simulink model "Pacemaker_Assignment2_group33"  (R2020a)
settings: Solver=FixedStepAuto  StartTime=0.0  StopTime=10.0  FixedStep=1e-3  RelTol=1e-3  EnableMultiTasking=on
undefined symbols (not defined in the file): D0, D1, D10, D11, D12, D13, D2, D3, D4, D5, D6, D7, D8, D9, magnitude, PTA0, PTA1, PTA2, PTB23, PTB9, PTC16, PTC17, PTC2, PTC3, PTC4, PTD0, PTD1, PTD2, PTD3
libraries: frdmk64flib x17, dspstat3 x1
settings Model: ExtModeTrigDuration=5  Creator=sxj  LastModifiedBy=sxj
settings OptimizationCC: EnhancedBackFolding=on  PassReuseOutputArgsAs=Individual arguments  ZeroExternalMemoryAtStartup=off  ZeroInternalMemoryAtStartup=off  MaxStackSize=64  OptimizeBlockOrder=speed  DifferentSizesBufferReuse=on  OptimizationCustomize=off  EfficientTunableParamExpr=on
settings DebuggingCC: ParameterTunabilityLossMsg=error
settings HardwareCC: ProdBitPerPointer=32  ProdBitPerSizeT=32  ProdBitPerPtrDiffT=32  ProdLargestAtomicInteger=Long  ProdLargestAtomicFloat=Double  ProdWordSize=32  ProdHWDeviceType=ARM Compatible->ARM Cortex
settings SFSimCC: MATLABDynamicMemAlloc=off
settings RTWCC: SystemTargetFile=ert.tlc  HardwareBoard=NXP FRDM-K64F  TemplateMakefile=ert_default_tmf  Toolchain=GNU Tools for ARM Embedded Processors
settings CodeAppCC: ForceParamTrailComments=on  IgnoreCustomStorageClasses=off  OperatorAnnotations=on  SimulinkDataObjDesc=on  SFDataObjDesc=on  InsertBlockDesc=on

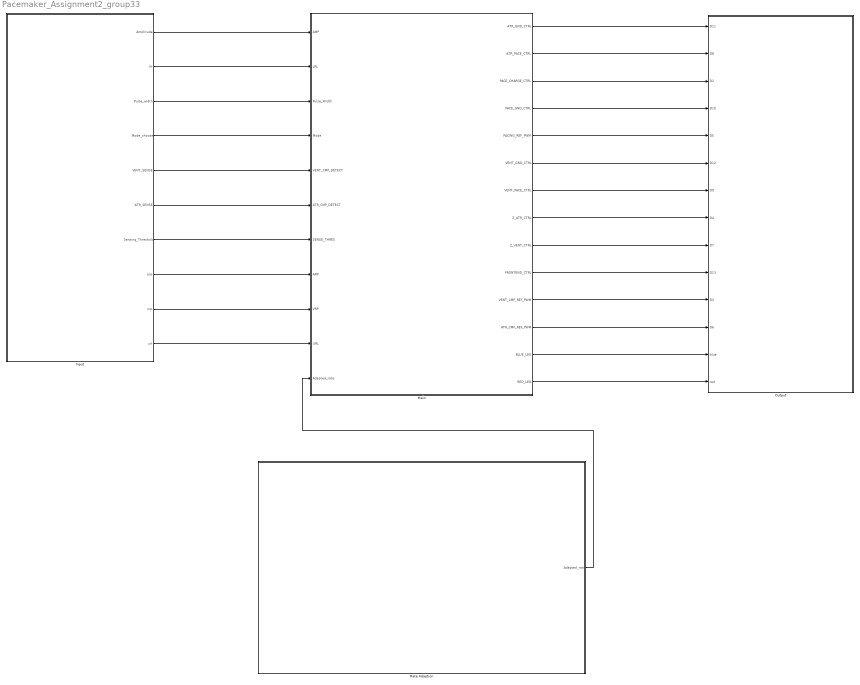
== system Pacemaker_Assignment2_group33 ==
  Input : Subsystem
  Main : Stateflow chart  TreatAsAtomicUnit=on
  Output : Subsystem
  Rate Adaption : Subsystem
  wires:
  Input/1(Amplitude) -> Main/1(AMP)
  Input/2(lrl) -> Main/2(LRL)
  Input/3(Pulse_width) -> Main/3(Pulse_Width)
  Input/4(Mode_choose) -> Main/4(Mode)
  Input/5(VENT_SENSE) -> Main/5(VENT_CMP_DETECT)
  Input/6(ATR_SENSE) -> Main/6(ATR_CMP_DETECT)
  Input/7(Sensing_Threshold) -> Main/7(SENSE_THRES)
  Main/1(ATR_GND_CTRL) -> Output/1(D11)
  Main/2(ATR_PACE_CTRL) -> Output/2(D8)
  Main/3(PACE_CHARGE_CTRL) -> Output/3(D2)
  Main/4(PACE_GND_CTRL) -> Output/4(D10)
  Main/5(PACING_REF_PWM) -> Output/5(D5)
  Main/6(VENT_GND_CTRL) -> Output/6(D12)
  Main/7(VENT_PACE_CTRL) -> Output/7(D9)
  Main/8(Z_ATR_CTRL) -> Output/8(D4)
  Main/9(Z_VENT_CTRL) -> Output/9(D7)
  Main/10(FRONTEND_CTRL) -> Output/10(D13)
  Main/11(VENT_CMP_REF_PWM) -> Output/11(D3)
  Main/12(ATR_CMP_REF_PWM) -> Output/12(D6)
  Main/13(BLUE_LED) -> Output/13(blue)
  Main/14(RED_LED) -> Output/14(red)
  Input/8(arp) -> Main/8(ARP)
  Input/9(vrp) -> Main/9(VRP)
  Input/10(url) -> Main/10(URL)
  Rate Adaption/1(Adapted_rate) -> Main/11(Adapted_rate)

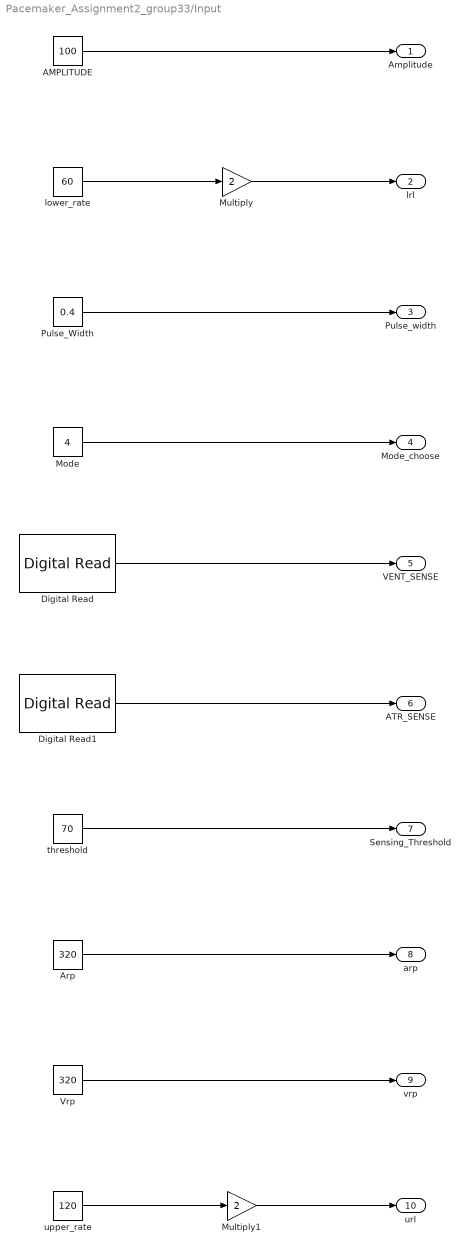
== system Pacemaker_Assignment2_group33/Input ==
  AMPLITUDE : Constant  Value=100
  Arp : Constant  Value=320
  Digital Read : frdmk64flib/Digital Read  Whichpin=PTC17 (D1)  SampleTime=-1
  Digital Read1 : frdmk64flib/Digital Read  Whichpin=PTC16 (D0)  SampleTime=-1
  Mode : Constant  Value=4
  Multiply : Gain  Gain=2
  Multiply1 : Gain  Gain=2
  Pulse_Width : Constant  Value=0.4
  Vrp : Constant  Value=320
  lower_rate : Constant  Value=60
  threshold : Constant  Value=70
  upper_rate : Constant  Value=120
  Amplitude : Outport
  lrl : Outport  Port=2
  Pulse_width : Outport  Port=3
  Mode_choose : Outport  Port=4
  VENT_SENSE : Outport  Port=5
  ATR_SENSE : Outport  Port=6
  Sensing_Threshold : Outport  Port=7
  arp : Outport  Port=8
  vrp : Outport  Port=9
  url : Outport  Port=10
  wires:
  AMPLITUDE/1 -> Amplitude/1
  Pulse_Width/1 -> Pulse_width/1
  Mode/1 -> Mode_choose/1
  Digital Read/1 -> VENT_SENSE/1
  Digital Read1/1 -> ATR_SENSE/1
  threshold/1 -> Sensing_Threshold/1
  Arp/1 -> arp/1
  Vrp/1 -> vrp/1
  lower_rate/1 -> Multiply/1
  Multiply/1 -> lrl/1
  upper_rate/1 -> Multiply1/1
  Multiply1/1 -> url/1

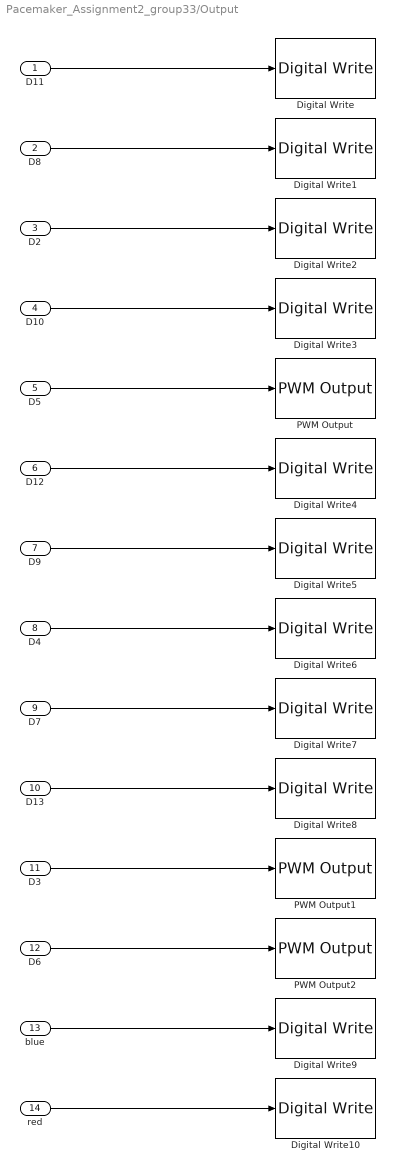
== system Pacemaker_Assignment2_group33/Output ==
  D11 : Inport
  D8 : Inport  Port=2
  D2 : Inport  Port=3
  D10 : Inport  Port=4
  D5 : Inport  Port=5
  D12 : Inport  Port=6
  D9 : Inport  Port=7
  D4 : Inport  Port=8
  D7 : Inport  Port=9
  D13 : Inport  Port=10
  D3 : Inport  Port=11
  D6 : Inport  Port=12
  blue : Inport  Port=13
  red : Inport  Port=14
  Digital Write : frdmk64flib/Digital Write  Whichpin=PTD2 (D11)
  Digital Write1 : frdmk64flib/Digital Write  Whichpin=PTA0 (D8)
  Digital Write10 : frdmk64flib/Digital Write  Whichpin=RED_LED
  Digital Write2 : frdmk64flib/Digital Write  Whichpin=PTB9 (D2)
  Digital Write3 : frdmk64flib/Digital Write  Whichpin=PTD0 (D10)
  Digital Write4 : frdmk64flib/Digital Write  Whichpin=PTD3 (D12)
  Digital Write5 : frdmk64flib/Digital Write  Whichpin=PTC4 (D9)
  Digital Write6 : frdmk64flib/Digital Write  Whichpin=PTB23 (D4)
  Digital Write7 : frdmk64flib/Digital Write  Whichpin=PTC3 (D7)
  Digital Write8 : frdmk64flib/Digital Write  Whichpin=PTD1 (D13)
  Digital Write9 : frdmk64flib/Digital Write  Whichpin=BLUE_LED
  PWM Output : frdmk64flib/PWM Output  Whichpin=PTA2 (D5)  InitialFrequency=2000  InitialDutyCycle=0
  PWM Output1 : frdmk64flib/PWM Output  Whichpin=PTA1 (D3)  InitialFrequency=2000  InitialDutyCycle=0
  PWM Output2 : frdmk64flib/PWM Output  Whichpin=PTC2 (D6)  InitialFrequency=2000  InitialDutyCycle=0
  wires:
  D11/1 -> Digital Write/1
  D8/1 -> Digital Write1/1
  D2/1 -> Digital Write2/1
  D10/1 -> Digital Write3/1
  D5/1 -> PWM Output/1
  D12/1 -> Digital Write4/1
  D9/1 -> Digital Write5/1
  D4/1 -> Digital Write6/1
  D7/1 -> Digital Write7/1
  D13/1 -> Digital Write8/1
  D3/1 -> PWM Output1/1
  D6/1 -> PWM Output2/1
  blue/1 -> Digital Write9/1
  red/1 -> Digital Write10/1

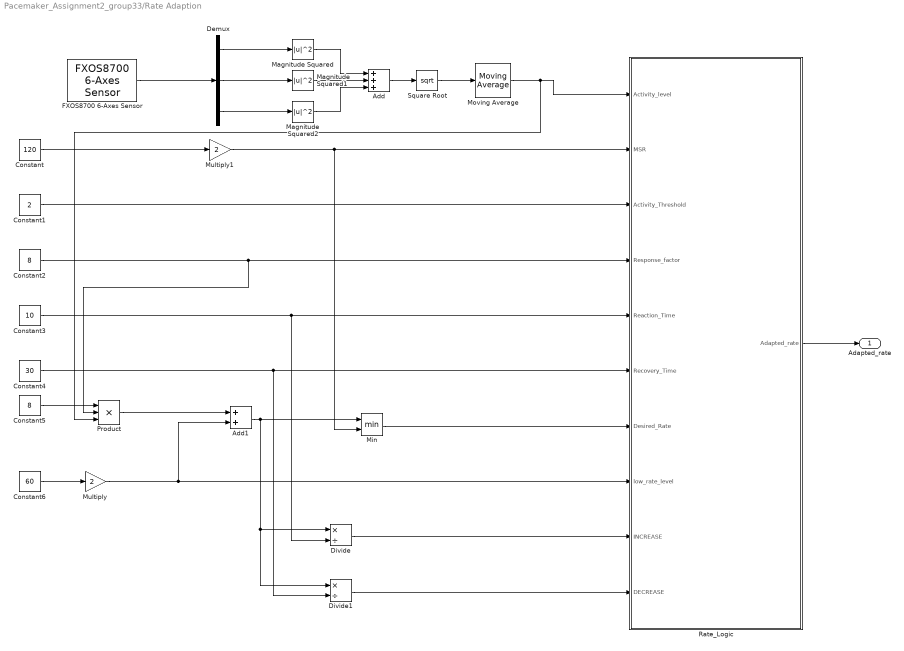
== system Pacemaker_Assignment2_group33/Rate Adaption ==
  Add : Sum  Inputs=+++
  Add1 : Sum
  Constant : Constant  Value=120
  Constant1 : Constant  Value=2
  Constant2 : Constant  Value=8
  Constant3 : Constant  Value=10
  Constant4 : Constant  Value=30
  Constant5 : Constant  Value=8
  Constant6 : Constant  Value=60
  Demux : Demux  Outputs=3
  Divide : Product  Inputs=*/
  Divide1 : Product  Inputs=*/
  FXOS8700 6-Axes Sensor : frdmk64flib/FXOS8700 6-Axes Sensor  Activesensor=Accelerometer only  ODR=800Hz  HybridODR=400Hz  Accelfullrange=-4g to +4g  SampleTime=-1
  Magnitude Squared : Math  Operator=magnitude^2  SaturateOnIntegerOverflow=on
  Magnitude Squared1 : Math  Operator=magnitude^2  SaturateOnIntegerOverflow=on
  Magnitude Squared2 : Math  Operator=magnitude^2  SaturateOnIntegerOverflow=on
  Min : MinMax  Inputs=2
  Moving Average : dspstat3/Moving Average  Method=Sliding window  ForgettingFactorPort=off  SpecifyWindowLength=on  WindowLength=100  ForgettingFactor=0.9  SimulateUsing=Code generation
  Multiply : Gain  Gain=2
  Multiply1 : Gain  Gain=2
  Product : Product  Inputs=3
  Rate_Logic : Stateflow chart  TreatAsAtomicUnit=on
  Square Root : Sqrt  SaturateOnIntegerOverflow=on
  Adapted_rate : Outport
  wires:
  Demux/1 -> Magnitude Squared/1
  Magnitude Squared1/1 -> Add/2
  Add/1 -> Square Root/1
  FXOS8700 6-Axes Sensor/1 -> Demux/1
  Demux/2 -> Magnitude Squared1/1
  Demux/3 -> Magnitude Squared2/1
  Magnitude Squared/1 -> Add/1
  Magnitude Squared2/1 -> Add/3
  Square Root/1 -> Moving Average/1
  Constant/1 -> Multiply1/1
  Constant1/1 -> Rate_Logic/3(Activity_Threshold)
  Constant2/1 -> Product/2, Rate_Logic/4(Response_factor)
  Constant3/1 -> Divide/2, Rate_Logic/5(Reaction_Time)
  Constant4/1 -> Divide1/2, Rate_Logic/6(Recovery_Time)
  Moving Average/1 -> Product/3, Rate_Logic/1(Activity_level)
  Product/1 -> Add1/1
  Multiply/1 -> Add1/2, Rate_Logic/8(low_rate_level)
  Add1/1 -> Divide1/1, Divide/1, Min/1
  Min/1 -> Rate_Logic/7(Desired_Rate)
  Divide/1 -> Rate_Logic/9(INCREASE)
  Rate_Logic/1(Adapted_rate) -> Adapted_rate/1
  Constant5/1 -> Product/1
  Divide1/1 -> Rate_Logic/10(DECREASE)
  Constant6/1 -> Multiply/1
  Multiply1/1 -> Min/2, Rate_Logic/2(MSR)

== stateflow chart Pacemaker_Assignment2_group33/Rate Adaption/Rate_Logic ==
  state Increase_pend
  state Initialize
    entry:
    Adapted_rate = low_rate_level;
  state Increase_
    entry:
    Adapted_rate = Adapted_rate + INCREASE;
  state Reached_desire
    entry:
    Adapted_rate = Desired_Rate;
  state Inc_Dec
  state Dec_Inc
  state Decrease_
    entry:
    Adapted_rate = Adapted_rate - DECREASE;
  state Decrease_pend
  Increase_pend -> Increase_ : after(1000,msec)
  Increase_ -> Increase_pend [order 1] : [Adapted_rate < Desired_Rate]
  (default) -> Initialize
  Initialize -> Initialize [order 2] : [Activity_level <= Activity_Threshold]
  Reached_desire -> Reached_desire [order 2] : [Activity_level > Activity_Threshold]
  Initialize -> Increase_ [order 1] : [Activity_level > Activity_Threshold]
  Increase_ -> Reached_desire [order 2] : [Adapted_rate >= Desired_Rate]
  Increase_ -> Inc_Dec [order 3] : [Activity_level <= Activity_Threshold]
  Dec_Inc -> Increase_ : after(1000,msec)
  Decrease_ -> Initialize [order 2] : [Adapted_rate <= low_rate_level]
  Reached_desire -> Decrease_ [order 1] : [Activity_level <= Activity_Threshold]
  Inc_Dec -> Decrease_ : after(1000,msec)
  Decrease_ -> Dec_Inc [order 1] : [Activity_level > Activity_Threshold]
  Decrease_ -> Decrease_pend [order 3] : [Adapted_rate > low_rate_level]
  Decrease_pend -> Decrease_ : after(1000,msec)
  data: Activity_level input; MSR input; Activity_Threshold input; Response_factor input; Reaction_Time input; Recovery_Time input; Desired_Rate input; low_rate_level input; INCREASE input; DECREASE input; Adapted_rate output

== stateflow chart Pacemaker_Assignment2_group33/Main ==
  state AOO
    state AOO_CHARGE
      %State for charging C22 and Discharging C21
      entry:
      PACING_REF_PWM = AMP;
      PACE_CHARGE_CTRL = 1;
      ATR_PACE_CTRL = 0;
      ATR_GND_CTRL = 1;
      PACE_GND_CTRL = 1;
      Z_ATR_CTRL = 0;
      VENT_PACE_CTRL = 0;
      VENT_GND_CTRL = 0;
      Z_VENT_CTRL = 0;
      BLUE_LED = 0;
      RED_LED = 0;
    state AOO_PACE
      %State for pacemaker actual pacing
      entry:
      PACING_REF_PWM = AMP;
      PACE_CHARGE_CTRL = 0;
      ATR_PACE_CTRL = 1;
      ATR_GND_CTRL = 0;
      PACE_GND_CTRL = 1;
      Z_ATR_CTRL = 0;
      VENT_PACE_CTRL = 0;
      VENT_GND_CTRL = 0;
      Z_VENT_CTRL = 0;
      BLUE_LED = 1;
      RED_LED = 0;
    (default) -> AOO_CHARGE
    AOO_CHARGE -> AOO_PACE : [after((60000/LRL)-Pulse_Width,msec)]
    AOO_PACE -> AOO_CHARGE : [after(Pulse_Width,msec)]
  state AOOR
    state AOOR_PACE
      %State for pacemaker actual pacing
      entry:
      PACING_REF_PWM = AMP;
      PACE_CHARGE_CTRL = 0;
      ATR_PACE_CTRL = 1;
      ATR_GND_CTRL = 0;
      PACE_GND_CTRL = 1;
      Z_ATR_CTRL = 0;
      VENT_PACE_CTRL = 0;
      VENT_GND_CTRL = 0;
      Z_VENT_CTRL = 0;
      BLUE_LED = 1;
      RED_LED = 0;
    state AOOR_CHARGE
      %State for charging C22 and Discharging C21
      entry:
      PACING_REF_PWM = AMP;
      PACE_CHARGE_CTRL = 1;
      ATR_PACE_CTRL = 0;
      ATR_GND_CTRL = 1;
      PACE_GND_CTRL = 1;
      Z_ATR_CTRL = 0;
      VENT_PACE_CTRL = 0;
      VENT_GND_CTRL = 0;
      Z_VENT_CTRL = 0;
      BLUE_LED = 0;
      RED_LED = 1;
    (default) -> AOOR_CHARGE
    AOOR_CHARGE -> AOOR_PACE : after(60000/Adapted_rate-Pulse_Width,msec)
    AOOR_PACE -> AOOR_CHARGE : after(Pulse_Width,msec)
  state VVIR
    state VVI_entry
      %Entry State setting variables
      % identical to Charging State
      entry:
      PACING_REF_PWM = AMP;
      PACE_CHARGE_CTRL = 1;
      VENT_PACE_CTRL = 0;
      VENT_GND_CTRL = 1;
      PACE_GND_CTRL = 1;
      Z_VENT_CTRL = 0;
      FRONTEND_CTRL = 1;
      VENT_CMP_REF_PWM = SENSE_THRES;
      ATR_PACE_CTRL = 0;
      ATR_GND_CTRL = 0;
      Z_ATR_CTRL = 0;
    state Sensed
      %Natural activities detected
    state VVI_CHARGE
      %State for charging C22 and Discharging C21
      entry:
      PACING_REF_PWM = AMP;
      PACE_CHARGE_CTRL = 1;
      VENT_PACE_CTRL = 0;
      VENT_GND_CTRL = 1;
      PACE_GND_CTRL = 1;
      Z_VENT_CTRL = 0;
      FRONTEND_CTRL = 1;
      VENT_CMP_REF_PWM = SENSE_THRES;
      ATR_PACE_CTRL = 0;
      ATR_GND_CTRL = 0;
      Z_ATR_CTRL = 0;
    state VVI_Sense
      %Detect Natural activities
    state VVI_PACE
      %State for pacamekr actual pacing
      entry:
      PACING_REF_PWM = AMP;
      PACE_CHARGE_CTRL = 0;
      VENT_PACE_CTRL = 1;
      VENT_GND_CTRL = 0;
      PACE_GND_CTRL = 1;
      Z_VENT_CTRL = 0;
      FRONTEND_CTRL = 1;
      VENT_CMP_REF_PWM = SENSE_THRES;
      ATR_PACE_CTRL = 0;
      ATR_GND_CTRL = 0;
      Z_ATR_CTRL = 0;
    (default) -> VVIR.VVI_entry
    VVIR.Sensed -> VVIR.VVI_Sense : after(VRP,msec)
    VVIR.VVI_entry -> VVIR.VVI_Sense
    VVIR.VVI_Sense -> VVIR.Sensed [order 1] : [VENT_CMP_DETECT == 1]
    VVIR.VVI_Sense -> VVIR.VVI_PACE [order 2] : after((60000/Adapted_rate)-VRP,msec)
    VVIR.VVI_CHARGE -> VVIR.VVI_Sense : after(VRP-Pulse_Width,msec)
    VVIR.VVI_PACE -> VVIR.VVI_CHARGE : after(Pulse_Width,msec)
  state IDLE_STATE
  state VVI
    state VVI_entry
      %Entry State setting variables
      % identical to Charging State
      entry:
      PACING_REF_PWM = AMP;
      PACE_CHARGE_CTRL = 1;
      VENT_PACE_CTRL = 0;
      VENT_GND_CTRL = 1;
      PACE_GND_CTRL = 1;
      Z_VENT_CTRL = 0;
      FRONTEND_CTRL = 1;
      VENT_CMP_REF_PWM = SENSE_THRES;
      ATR_PACE_CTRL = 0;
      ATR_GND_CTRL = 0;
      Z_ATR_CTRL = 0;
    state Sensed
      %Natural activities detected
    state VVI_CHARGE
      %State for charging C22 and Discharging C21
      entry:
      PACING_REF_PWM = AMP;
      PACE_CHARGE_CTRL = 1;
      VENT_PACE_CTRL = 0;
      VENT_GND_CTRL = 1;
      PACE_GND_CTRL = 1;
      Z_VENT_CTRL = 0;
      FRONTEND_CTRL = 1;
      VENT_CMP_REF_PWM = SENSE_THRES;
      ATR_PACE_CTRL = 0;
      ATR_GND_CTRL = 0;
      Z_ATR_CTRL = 0;
    state VVI_Sense
      %Detect Natural activities
    state VVI_PACE
      %State for pacamekr actual pacing
      entry:
      PACING_REF_PWM = AMP;
      PACE_CHARGE_CTRL = 0;
      VENT_PACE_CTRL = 1;
      VENT_GND_CTRL = 0;
      PACE_GND_CTRL = 1;
      Z_VENT_CTRL = 0;
      FRONTEND_CTRL = 1;
      VENT_CMP_REF_PWM = SENSE_THRES;
      ATR_PACE_CTRL = 0;
      ATR_GND_CTRL = 0;
      Z_ATR_CTRL = 0;
    (default) -> VVI.VVI_entry
    VVI.Sensed -> VVI.VVI_Sense : after(VRP,msec)
    VVI.VVI_entry -> VVI.VVI_Sense
    VVI.VVI_Sense -> VVI.Sensed [order 1] : [VENT_CMP_DETECT == 1]
    VVI.VVI_Sense -> VVI.VVI_PACE [order 2] : after((60000/LRL)-VRP,msec)
    VVI.VVI_CHARGE -> VVI.VVI_Sense : after(VRP-Pulse_Width,msec)
    VVI.VVI_PACE -> VVI.VVI_CHARGE : after(Pulse_Width,msec)
  state AAI
    state AAI_entry
      %Entry State setting variables
      % identical to Charging State
      entry:
      PACING_REF_PWM = AMP;
      PACE_CHARGE_CTRL = 1;
      ATR_PACE_CTRL = 0;
      ATR_GND_CTRL = 1;
      PACE_GND_CTRL = 1;
      Z_ATR_CTRL = 0;
      FRONTEND_CTRL = 1;
      ATR_CMP_REF_PWM = SENSE_THRES;
      VENT_PACE_CTRL = 0;
      VENT_GND_CTRL = 0;
      Z_VENT_CTRL = 0;
    state AAI_Sensed
      %Nastural actvites Detected
    state AAI_PACE
      %State for pacamekr actual pacing
      entry:
      PACING_REF_PWM = AMP;
      PACE_CHARGE_CTRL = 0;
      ATR_PACE_CTRL = 1;
      ATR_GND_CTRL = 0;
      PACE_GND_CTRL = 1;
      Z_ATR_CTRL = 0;
      FRONTEND_CTRL = 1;
      ATR_CMP_REF_PWM = SENSE_THRES;
      VENT_PACE_CTRL = 0;
      VENT_GND_CTRL = 0;
      Z_VENT_CTRL = 0;
    state AAI_CHARGE
      %State for charging C22 and Discharging C21
      entry:
      PACING_REF_PWM = AMP;
      PACE_CHARGE_CTRL = 1;
      ATR_PACE_CTRL = 0;
      ATR_GND_CTRL = 1;
      PACE_GND_CTRL = 1;
      Z_ATR_CTRL = 0;
      FRONTEND_CTRL = 1;
      ATR_CMP_REF_PWM = SENSE_THRES;
      VENT_PACE_CTRL = 0;
      VENT_GND_CTRL = 0;
      Z_VENT_CTRL = 0;
    state AAI_Sense
      %Detect Natural activities
    (default) -> AAI.AAI_entry
    AAI.AAI_entry -> AAI.AAI_Sense
    AAI.AAI_Sensed -> AAI.AAI_Sense : after(ARP,msec)
    AAI.AAI_Sense -> AAI.AAI_Sensed [order 1] : [ATR_CMP_DETECT == 1]
    AAI.AAI_CHARGE -> AAI.AAI_Sense : after(ARP-Pulse_Width,msec)
    AAI.AAI_Sense -> AAI.AAI_PACE [order 2] : after((60000/LRL)-ARP,msec)
    AAI.AAI_PACE -> AAI.AAI_CHARGE : after(Pulse_Width,msec)
  state AAIR
    state AAI_entry
      %Entry State setting variables
      % identical to Charging State
      entry:
      PACING_REF_PWM = AMP;
      PACE_CHARGE_CTRL = 1;
      ATR_PACE_CTRL = 0;
      ATR_GND_CTRL = 1;
      PACE_GND_CTRL = 1;
      Z_ATR_CTRL = 0;
      FRONTEND_CTRL = 1;
      ATR_CMP_REF_PWM = SENSE_THRES;
      VENT_PACE_CTRL = 0;
      VENT_GND_CTRL = 0;
      Z_VENT_CTRL = 0;
    state AAI_Sensed
      %Nastural actvites Detected
    state AAI_PACE
      %State for pacamekr actual pacing
      entry:
      PACING_REF_PWM = AMP;
      PACE_CHARGE_CTRL = 0;
      ATR_PACE_CTRL = 1;
      ATR_GND_CTRL = 0;
      PACE_GND_CTRL = 1;
      Z_ATR_CTRL = 0;
      FRONTEND_CTRL = 1;
      ATR_CMP_REF_PWM = SENSE_THRES;
      VENT_PACE_CTRL = 0;
      VENT_GND_CTRL = 0;
      Z_VENT_CTRL = 0;
    state AAI_CHARGE
      %State for charging C22 and Discharging C21
      entry:
      PACING_REF_PWM = AMP;
      PACE_CHARGE_CTRL = 1;
      ATR_PACE_CTRL = 0;
      ATR_GND_CTRL = 1;
      PACE_GND_CTRL = 1;
      Z_ATR_CTRL = 0;
      FRONTEND_CTRL = 1;
      ATR_CMP_REF_PWM = SENSE_THRES;
      VENT_PACE_CTRL = 0;
      VENT_GND_CTRL = 0;
      Z_VENT_CTRL = 0;
    state AAI_Sense
      %Detect Natural activities
    (default) -> AAIR.AAI_entry
    AAIR.AAI_entry -> AAIR.AAI_Sense
    AAIR.AAI_Sensed -> AAIR.AAI_Sense : after(ARP,msec)
    AAIR.AAI_Sense -> AAIR.AAI_Sensed [order 1] : [ATR_CMP_DETECT == 1]
    AAIR.AAI_CHARGE -> AAIR.AAI_Sense : after(ARP-Pulse_Width,msec)
    AAIR.AAI_Sense -> AAIR.AAI_PACE [order 2] : after((60000/Adapted_rate)-ARP,msec)
    AAIR.AAI_PACE -> AAIR.AAI_CHARGE : after(Pulse_Width,msec)
  state VOOR
    state VOO_PACE
      %State for pacemaker actual pacing
      entry:
      PACING_REF_PWM = AMP;
      PACE_CHARGE_CTRL = 0;
      VENT_PACE_CTRL = 1;
      VENT_GND_CTRL = 0;
      PACE_GND_CTRL = 1;
      Z_VENT_CTRL = 0;
      ATR_PACE_CTRL = 0;
      ATR_GND_CTRL = 0;
      Z_ATR_CTRL = 0;
      BLUE_LED = 1;
      RED_LED = 0;
    state VOO_CHARGE
      %State for charging C22 and Discharging C21
      entry:
      PACING_REF_PWM = AMP;
      PACE_CHARGE_CTRL = 1;
      VENT_PACE_CTRL = 0;
      VENT_GND_CTRL = 1;
      PACE_GND_CTRL = 1;
      Z_VENT_CTRL = 0;
      ATR_PACE_CTRL = 0;
      ATR_GND_CTRL = 0;
      Z_ATR_CTRL = 0;
      BLUE_LED = 0;
      RED_LED = 1;
    (default) -> VOOR.VOO_CHARGE
    VOOR.VOO_CHARGE -> VOOR.VOO_PACE : after(60000/Adapted_rate-Pulse_Width,msec)
    VOOR.VOO_PACE -> VOOR.VOO_CHARGE : after(Pulse_Width,msec)
  state VOO
    state VOO_CHARGE
      %State for charging C22 and Discharging C21
      entry:
      PACING_REF_PWM = AMP;
      PACE_CHARGE_CTRL = 1;
      VENT_PACE_CTRL = 0;
      VENT_GND_CTRL = 1;
      PACE_GND_CTRL = 1;
      Z_VENT_CTRL = 0;
      ATR_PACE_CTRL = 0;
      ATR_GND_CTRL = 0;
      Z_ATR_CTRL = 0;
      BLUE_LED = 0;
      RED_LED = 0;
    state VOO_PACE
      %State for pacemaker actual pacing
      entry:
      PACING_REF_PWM = AMP;
      PACE_CHARGE_CTRL = 0;
      VENT_PACE_CTRL = 1;
      VENT_GND_CTRL = 0;
      PACE_GND_CTRL = 1;
      Z_VENT_CTRL = 0;
      ATR_PACE_CTRL = 0;
      ATR_GND_CTRL = 0;
      Z_ATR_CTRL = 0;
      BLUE_LED = 1;
      RED_LED = 0;
    (default) -> VOO.VOO_CHARGE
    VOO.VOO_CHARGE -> VOO.VOO_PACE : after((60000/LRL)-Pulse_Width,msec)
    VOO.VOO_PACE -> VOO.VOO_CHARGE : after(Pulse_Width,msec)
  IDLE_STATE -> AOO [order 1] : [Mode == 0]
  AOO -> IDLE_STATE : [Mode ~= 0]
  IDLE_STATE -> AOOR [order 5] : [Mode == 4]
  AOOR -> IDLE_STATE : [Mode ~= 4]
  IDLE_STATE -> VVIR [order 8] : [Mode == 7]
  VVIR -> IDLE_STATE : [Mode ~= 7]
  (default) -> IDLE_STATE
  IDLE_STATE -> VVI [order 4] : [Mode == 3]
  IDLE_STATE -> AAI [order 3] : [Mode == 2]
  AAI -> IDLE_STATE : [Mode ~= 2]
  VVI -> IDLE_STATE : [Mode ~= 3]
  IDLE_STATE -> AAIR [order 7] : [Mode == 6]
  AAIR -> IDLE_STATE : [Mode ~= 6]
  IDLE_STATE -> VOOR [order 6] : [Mode == 5]
  IDLE_STATE -> VOO [order 2] : [Mode == 1]
  VOO -> IDLE_STATE : [Mode ~= 1]
  VOOR -> IDLE_STATE : [Mode ~= 5]
  data: AMP input; ATR_GND_CTRL output; ATR_PACE_CTRL output; PACE_CHARGE_CTRL output; PACE_GND_CTRL output; PACING_REF_PWM output; VENT_GND_CTRL output; VENT_PACE_CTRL output; Z_ATR_CTRL output; Z_VENT_CTRL output; LRL input; Pulse_Width input; Mode input; FRONTEND_CTRL output; VENT_CMP_DETECT input; ATR_CMP_DETECT input; SENSE_THRES input; VENT_CMP_REF_PWM output; ATR_CMP_REF_PWM output; BLUE_LED output; RED_LED output; ARP input; VRP input; URL input; Adapted_rate input
